simulink model "multi_PMSGs_github"  (R2024a)
settings: Solver=ode1  StartTime=0.0  StopTime=0.5  RelTol=1e-3  EnableMultiTasking=on
libraries: spsCurrentMeasurementLib x3, spsVoltageMeasurementLib x3, spsSeriesRLCBranchLib x2, eeGeneralControl x2, simulink x2, spsdq0toabcLib x2, spsPermanentMagnetSynchronousMachineLib x2, spsUniversalBridgeLib x2, spsGroundLib x1, sps_lib x1
settings Model: Creator=Ruochen Zhao  LastModifiedBy=赵若辰
settings SolverCC: AllowMultiTaskInputOutput=on  PositivePriorityOrder=on  AutoInsertRateTranBlk=on

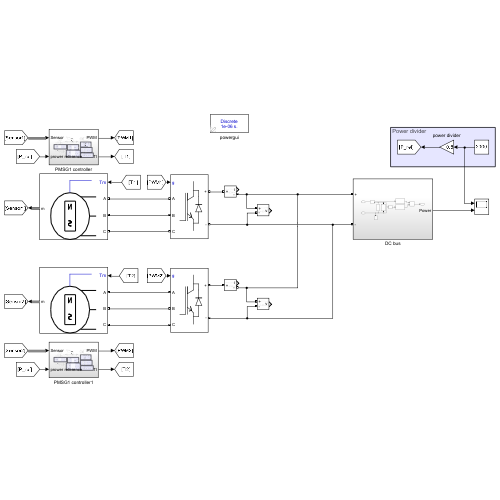
[thumbnail: Simulink's stored preview of the top-level diagram]
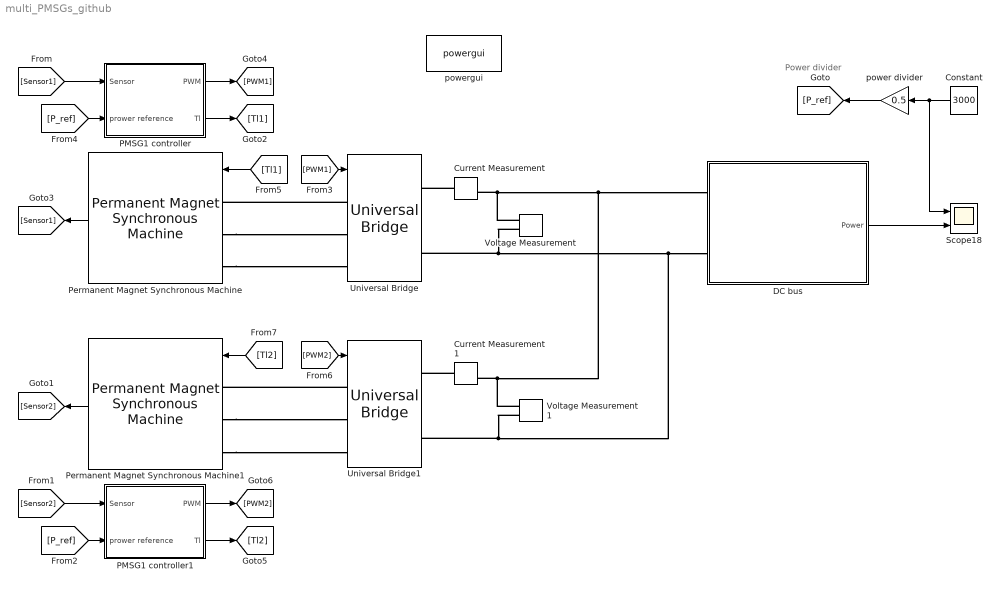
== system multi_PMSGs_github ==
  note: Power divider
  Constant : Constant  Value=3000
  Current Measurement : spsCurrentMeasurementLib/Current Measurement  PhasorSimulation=off  OutputType=Complex  PSBequivalent=0
  Current Measurement1 : spsCurrentMeasurementLib/Current Measurement  PhasorSimulation=off  OutputType=Complex  PSBequivalent=0
  DC bus : Subsystem
  PMSG1 controller : Subsystem
  PMSG1 controller1 : Subsystem
  Permanent Magnet Synchronous Machine : spsPermanentMagnetSynchronousMachineLib/Permanent Magnet Synchronous Machine  NbPhases=3  FluxDistribution=Sinusoidal  RotorType=Salient-pole  MechanicalLoad=Torque Tm  PresetModel=No  ShowDetailedParameters=on  MeasurementBus=off  Resistance=1.3  Inductance=8.5e-3  dqInductances=[0.75e-3,0.75e-3]  La=0.75e-3  MachineConstant=Flux linkage established by magnets (V.s)  Flux=0.4  VoltageCst=145.1039  TorqueCst=1.2  Flat=120  Mechanical="[0.0008 0.00001  2 0 ]"  PolePairs=4  InitialConditions=[0,0, 0,0]  InitialConditions5ph=[0 0 0 0 0 0]  RefAngle=90 degrees behind phase A axis (modified Park)  IterativeDiscreteModel=Trapezoidal non iterative  TsBlock=-1  TsPowergui=0
  Permanent Magnet Synchronous Machine1 : spsPermanentMagnetSynchronousMachineLib/Permanent Magnet Synchronous Machine  NbPhases=3  FluxDistribution=Sinusoidal  RotorType=Salient-pole  MechanicalLoad=Torque Tm  PresetModel=No  ShowDetailedParameters=on  MeasurementBus=off  Resistance=1.3  Inductance=8.5e-3  dqInductances=[0.75e-3,0.75e-3]  La=0.75e-3  MachineConstant=Flux linkage established by magnets (V.s)  Flux=0.4  VoltageCst=145.1039  TorqueCst=1.2  Flat=120  Mechanical="[0.0008 0.00001  2 0 ]"  PolePairs=4  InitialConditions=[0,0, 0,0]  InitialConditions5ph=[0 0 0 0 0 0]  RefAngle=90 degrees behind phase A axis (modified Park)  IterativeDiscreteModel=Trapezoidal non iterative  TsBlock=-1  TsPowergui=0
  Scope18 : Scope  NumInputPorts=2
  Universal Bridge : spsUniversalBridgeLib/Universal Bridge  Arms=3  SnubberResistance=1e5  SnubberCapacitance=inf  Device=IGBT / Diodes  Ron=1e-3  Lon=0  ForwardVoltages="[  0  0  ]"  ForwardVoltage=0  GTOparameters=[ 10e-6 , 20e-6 ]  IGBTparameters=[ 1e-6 , 2e-6 ]  Measurements=None  Measurements_2=None  converterType=Rectifier
  Universal Bridge1 : spsUniversalBridgeLib/Universal Bridge  Arms=3  SnubberResistance=1e5  SnubberCapacitance=inf  Device=IGBT / Diodes  Ron=1e-3  Lon=0  ForwardVoltages="[  0  0  ]"  ForwardVoltage=0  GTOparameters=[ 10e-6 , 20e-6 ]  IGBTparameters=[ 1e-6 , 2e-6 ]  Measurements=None  Measurements_2=None  converterType=Rectifier
  Voltage Measurement : spsVoltageMeasurementLib/Voltage Measurement  PhasorSimulation=off  OutputType=Complex  PSBequivalent=0
  Voltage Measurement1 : spsVoltageMeasurementLib/Voltage Measurement  PhasorSimulation=off  OutputType=Complex  PSBequivalent=0
  power divider : Gain  Gain=0.5
  powergui : sps_lib/powergui  Priority=1  SimulationMode=Discrete  SampleTime=1e-6  frequency=60  Iterations=50  frequencyindice=0  Pbase=100e6  ErrMax=1e-4  UnitsV=kV  UnitsW=MW  buscounter=0  FunctionMessages=off  echomessages=off  EnableUseOfTLC=off  CurrentSourceSwitches=off  DisableSnubberDevices=off  DisableRonSwitches=off  DisableVfSwitches=off  DisplayEquations=off  AutomaticDiscreteSolvers=off  SolverType=Tustin/Backward Euler (TBE)  Interpol=off  ExternalGateDelay=off  methode=off  Ts=100  x0status=blocks  SPID=on  SwTol=0  HookPort=off  NonlinearTolerance=1e-4  nMaxIteration=100  ContinueOnMaxIteration=off  RestoreLinks=warning  ResistiveCurrentMeasurement=off  Frange=[0:2:500]  Ylog=off  Xlog=on  ShowGrid=off  save=off  variable=ZData  structure=0  ZoomFFT=off  StartTime=0.0  cycles=1  DisplayStyle=1  fundamental=60  FreqAxis=off  MaxFrequency=1000  frequencyindicesteady=1  RmsSteady=1  display=off
  wires:
  Permanent Magnet Synchronous Machine/1 -> [Sensor1]
  [Tl1] -> Permanent Magnet Synchronous Machine/1
  [PWM1] -> Universal Bridge/1
  Permanent Magnet Synchronous Machine1/1 -> [Sensor2]
  [PWM2] -> Universal Bridge1/1
  [Sensor1] -> PMSG1 controller/1(Sensor)
  [P_ref] -> PMSG1 controller/2(prower reference)
  Constant/1 -> Scope18/1, power divider/1
  power divider/1 -> [P_ref]
  DC bus/1(Power) -> Scope18/2
  PMSG1 controller/2(Tl) -> [Tl1]
  PMSG1 controller/1(PWM) -> [PWM1]
  PMSG1 controller1/1(PWM) -> [PWM2]
  [P_ref] -> PMSG1 controller1/2(prower reference)
  [Sensor2] -> PMSG1 controller1/1(Sensor)
  PMSG1 controller1/2(Tl) -> [Tl2]
  [Tl2] -> Permanent Magnet Synchronous Machine1/1
  connections:
  Current Measurement1/RConn1 -- DC bus/LConn1 -- Voltage Measurement/LConn1 -- Current Measurement/RConn1 -- Voltage Measurement1/LConn1
  Universal Bridge1/RConn2 -- DC bus/LConn2 -- Voltage Measurement/LConn2 -- Universal Bridge/RConn2 -- Voltage Measurement1/LConn2
  Current Measurement/LConn1 -- Universal Bridge/RConn1
  Permanent Magnet Synchronous Machine/LConn3 -- Universal Bridge/LConn3
  Permanent Magnet Synchronous Machine/LConn2 -- Universal Bridge/LConn2
  Universal Bridge/LConn1 -- Permanent Magnet Synchronous Machine/LConn1
  Current Measurement1/LConn1 -- Universal Bridge1/RConn1
  Permanent Magnet Synchronous Machine1/LConn3 -- Universal Bridge1/LConn3
  Permanent Magnet Synchronous Machine1/LConn2 -- Universal Bridge1/LConn2
  Universal Bridge1/LConn1 -- Permanent Magnet Synchronous Machine1/LConn1

== system multi_PMSGs_github/DC bus ==
  Current Measurement : spsCurrentMeasurementLib/Current Measurement  PhasorSimulation=off  OutputType=Complex  PSBequivalent=0
  Ground : spsGroundLib/Ground  LConnTagsString=a
  Product : Product
  Series RLC Branch : spsSeriesRLCBranchLib/Series RLC Branch  LConnTagsString=__new0  RConnTagsString=__new0  BranchType=R  Resistance=10  Inductance=1e-3  SetiL0=off  InitialCurrent=0  Capacitance=200e-6  Setx0=off  InitialVoltage=0  Measurements=None
  Series RLC Branch1 : spsSeriesRLCBranchLib/Series RLC Branch  LConnTagsString=__new0  RConnTagsString=__new0  BranchType=C  Resistance=50  Inductance=1e-3  SetiL0=off  InitialCurrent=0  Capacitance=200e-6  Setx0=off  InitialVoltage=0  Measurements=None
  Transfer Fcn : TransferFcn  Numerator=[100]  Denominator=[1 100]
  Transfer Fcn1 : TransferFcn  Numerator=[100]  Denominator=[1 100]
  Voltage Measurement : spsVoltageMeasurementLib/Voltage Measurement  PhasorSimulation=off  OutputType=Complex  PSBequivalent=0
  + : PMIOPort  Side=Left
  - : PMIOPort  Port=2  Side=Left
  Power : Outport
  wires:
  Current Measurement/1 -> Transfer Fcn/1
  Transfer Fcn/1 -> Product/1
  Product/1 -> Power/1
  Voltage Measurement/1 -> Transfer Fcn1/1
  Transfer Fcn1/1 -> Product/2
  connections:
  Ground/LConn1 -- -/RConn1 -- Series RLC Branch1/RConn1 -- Voltage Measurement/LConn2 -- Series RLC Branch/RConn1
  Series RLC Branch/LConn1 -- Series RLC Branch1/LConn1 -- Voltage Measurement/LConn1 -- Current Measurement/RConn1
  Current Measurement/LConn1 -- +/RConn1

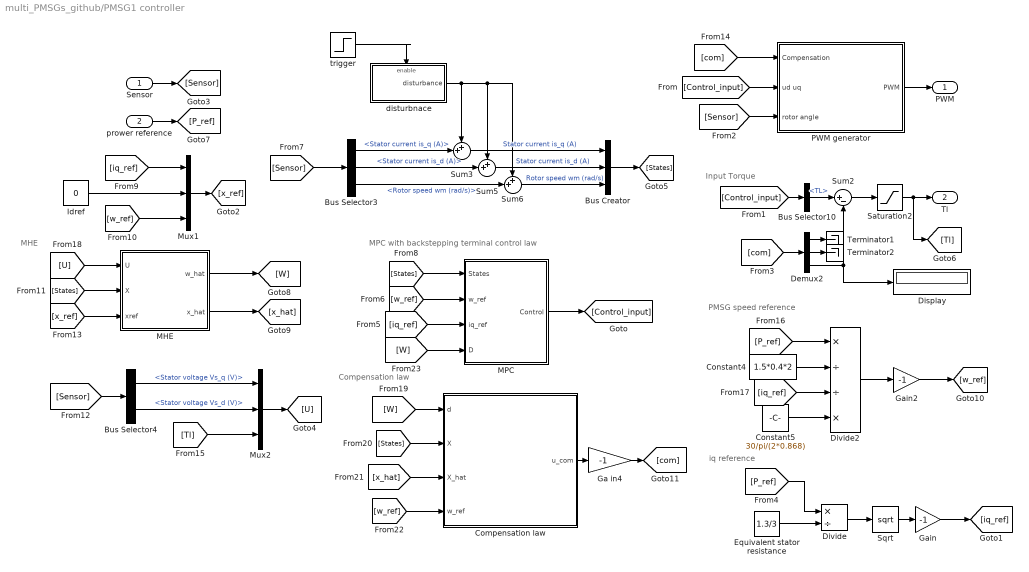
== system multi_PMSGs_github/PMSG1 controller ==
  note: MHE
  note: Compensation law
  note: iq reference
  note: PMSG speed reference
  note: MPC with backstepping terminal control law
  note: Input Torque
  Sensor : Inport
  prower reference : Inport  Port=2
  Bus Creator : BusCreator  Inputs=Stator current is_q (A),Stator current is_d (A),Rotor speed wm (rad/s)
  Bus Selector10 : BusSelector  OutputSignals=TL
  Bus Selector3 : BusSelector  OutputSignals=Stator current is_q (A),Stator current is_d (A),Rotor speed wm (rad/s)
  Bus Selector4 : BusSelector  OutputSignals=Stator voltage Vs_q (V),Stator voltage Vs_d (V)
  Compensation law : Subsystem  mask{K1=10000*10, K2=10000*6, K3=0}
      mask DialogControl ParameterGroupVar Prompt: 参数
  Constant4 : Constant  Value=1.5*0.4*2
  Constant5 : Constant  Value=30/pi/(2*0.868)
  Demux2 : Demux  Outputs=3
  Display : Display
  Divide : Product  Inputs=*/
  Divide2 : Product  Inputs=*//*
  Equivalent stator resistance : Constant  Value=1.3/3
  Ga in4 : Gain  Gain=-1
  Gain : Gain  Gain=-1
  Gain2 : Gain  Gain=-1
  Idref : Constant  Value=0
  MHE : Subsystem
  MPC : Subsystem  mask{q1=100, q2=100, q3=100, r1=0.01, r2=0.001, r3=0.001, N=10, K1=1e5*0.1, K2=1e5*0.1, K3=1e5*0.1, fc=100, Ts=1e-5}
      mask DialogControl DescGroupVar Prompt: MPC controller
      mask DialogControl ParameterGroupVar Prompt: Output Weight
      mask DialogControl Container3 Prompt: Input Weight
      mask DialogControl Container4 Prompt: Prediction Horizon
      mask DialogControl Container5 Prompt: Backstepping
      mask DialogControl Container6 Prompt: Filter
      mask DialogControl Container7 Prompt: Simple Time
  Mux1 : Mux  Inputs=3
  Mux2 : Mux  Inputs=3
  PWM generator : Subsystem
  Saturation2 : Saturate  UpperLimit=300  LowerLimit=-300
  Sqrt : Sqrt
  Sum2 : Sum  Inputs=|+-
  Sum3 : Sum  Inputs=++|
  Sum5 : Sum  Inputs=++|
  Sum6 : Sum  Inputs=++|
  Terminator1 : Terminator
  Terminator2 : Terminator
  disturbnace : Subsystem  mask{w1=50, A1=5, w2=100, A2=2, w3=150, A3=1}
      mask prompts: w1 "Frequency 1"; A1 "Amplitude 1"; w2 "Frequency 2"; A2 "Amplitude 2"; w3 "Frequency 3"; A3 "Amplitude 3"
      mask DialogControl ParameterGroupVar Prompt: 参数
  trigger : Step  Time=0.2  SampleTime=0
  PWM : Outport
  Tl : Outport  Port=2
  wires:
  Sensor/1 -> [Sensor]
  MPC/1(Control) -> [Control_input]
  [Control_input] -> Bus Selector10/1
  Bus Selector10/1 -> Sum2/1  "<TL>"
  Sum2/1 -> Saturation2/1
  [com] -> Demux2/1
  Demux2/3 -> Sum2/2, Display/1
  Demux2/1 -> Terminator1/1
  Demux2/2 -> Terminator2/1
  prower reference/1 -> [P_ref]
  Divide/1 -> Sqrt/1
  Equivalent stator resistance/1 -> Divide/2
  Sqrt/1 -> Gain/1
  [P_ref] -> Divide/1
  Gain/1 -> [iq_ref]
  [iq_ref] -> MPC/3(iq_ref)
  Bus Selector3/3 -> Sum6/2  "<Rotor speed wm (rad/s)>"
  Sum5/1 -> Bus Creator/2  "Stator current is_d (A)"
  Sum3/1 -> Bus Creator/1  "Stator current is_q (A)"
  Sum6/1 -> Bus Creator/3  "Rotor speed wm (rad/s)"
  Bus Selector3/1 -> Sum3/2  "<Stator current is_q (A)>"
  [Sensor] -> Bus Selector3/1
  Bus Selector3/2 -> Sum5/2  "<Stator current is_d (A)>"
  Bus Creator/1 -> [States]
  [com] -> PWM generator/1(Compensation)
  [Control_input] -> PWM generator/2(ud uq)
  [Sensor] -> PWM generator/3(rotor angle)
  PWM generator/1(PWM) -> PWM/1
  [iq_ref] -> Divide2/3
  Constant5/1 -> Divide2/4
  Gain2/1 -> [w_ref]
  Divide2/1 -> Gain2/1
  [P_ref] -> Divide2/1
  Constant4/1 -> Divide2/2
  [w_ref] -> MPC/2(w_ref)
  [States] -> MPC/1(States)
  disturbnace/1(disturbance) -> Sum6/1, Sum5/1, Sum3/1
  trigger/1 -> disturbnace/Enable
  [iq_ref] -> Mux1/1
  Idref/1 -> Mux1/2
  [w_ref] -> Mux1/3
  Mux1/1 -> [x_ref]
  [Tl] -> Mux2/3
  [Sensor] -> Bus Selector4/1
  Bus Selector4/2 -> Mux2/2  "<Stator voltage Vs_d (V)>"
  Mux2/1 -> [U]
  Bus Selector4/1 -> Mux2/1  "<Stator voltage Vs_q (V)>"
  [U] -> MHE/1("U ")
  [States] -> MHE/2(X)
  [x_ref] -> MHE/3(xref)
  MHE/1(w_hat) -> [W]
  [W] -> Compensation law/1(d)
  [States] -> Compensation law/2(X)
  MHE/2(x_hat) -> [x_hat]
  [x_hat] -> Compensation law/3(X_hat)
  [w_ref] -> Compensation law/4(w_ref)
  Ga in4/1 -> [com]
  Compensation law/1(u_com) -> Ga in4/1
  [W] -> MPC/4(D)
  Saturation2/1 -> [Tl], Tl/1

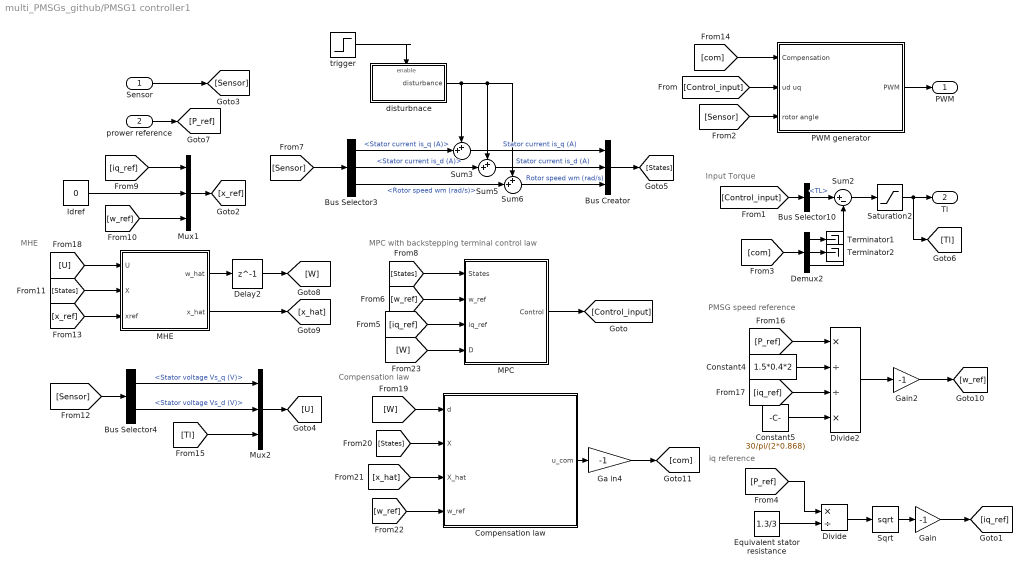
== system multi_PMSGs_github/PMSG1 controller1 ==
  note: MHE
  note: Compensation law
  note: iq reference
  note: PMSG speed reference
  note: MPC with backstepping terminal control law
  note: Input Torque
  Sensor : Inport
  prower reference : Inport  Port=2
  Bus Creator : BusCreator  Inputs=Stator current is_q (A),Stator current is_d (A),Rotor speed wm (rad/s)
  Bus Selector10 : BusSelector  OutputSignals=TL
  Bus Selector3 : BusSelector  OutputSignals=Stator current is_q (A),Stator current is_d (A),Rotor speed wm (rad/s)
  Bus Selector4 : BusSelector  OutputSignals=Stator voltage Vs_q (V),Stator voltage Vs_d (V)
  Compensation law : Subsystem  mask{K1=10000*10, K2=10000*6, K3=0}
      mask DialogControl ParameterGroupVar Prompt: 参数
  Constant4 : Constant  Value=1.5*0.4*2
  Constant5 : Constant  Value=30/pi/(2*0.868)
  Delay2 : Delay  DelayLength=1  InitialCondition=[0 0 0]
  Demux2 : Demux  Outputs=3
  Divide : Product  Inputs=*/
  Divide2 : Product  Inputs=*//*
  Equivalent stator resistance : Constant  Value=1.3/3
  Ga in4 : Gain  Gain=-1
  Gain : Gain  Gain=-1
  Gain2 : Gain  Gain=-1
  Idref : Constant  Value=0
  MHE : Subsystem
  MPC : Subsystem  mask{q1=100, q2=100, q3=100, r1=0.01, r2=0.001, r3=0.001, N=10, K1=1e5*0.1, K2=1e5*0.1, K3=1e5*0.1, fc=100, Ts=1e-5}
      mask DialogControl DescGroupVar Prompt: MPC controller
      mask DialogControl ParameterGroupVar Prompt: Output Weight
      mask DialogControl Container3 Prompt: Input Weight
      mask DialogControl Container4 Prompt: Prediction Horizon
      mask DialogControl Container5 Prompt: Backstepping
      mask DialogControl Container6 Prompt: Filter
      mask DialogControl Container7 Prompt: Simple Time
  Mux1 : Mux  Inputs=3
  Mux2 : Mux  Inputs=3
  PWM generator : Subsystem
  Saturation2 : Saturate  UpperLimit=300  LowerLimit=-300
  Sqrt : Sqrt
  Sum2 : Sum  Inputs=|+-
  Sum3 : Sum  Inputs=++|
  Sum5 : Sum  Inputs=++|
  Sum6 : Sum  Inputs=++|
  Terminator1 : Terminator
  Terminator2 : Terminator
  disturbnace : Subsystem  mask{w1=50, A1=5, w2=100, A2=2, w3=150, A3=1}
      mask prompts: w1 "Frequency 1"; A1 "Amplitude 1"; w2 "Frequency 2"; A2 "Amplitude 2"; w3 "Frequency 3"; A3 "Amplitude 3"
      mask DialogControl ParameterGroupVar Prompt: 参数
  trigger : Step  Time=0.2  After=0  SampleTime=0
  PWM : Outport
  Tl : Outport  Port=2
  wires:
  Sensor/1 -> [Sensor]
  MPC/1(Control) -> [Control_input]
  [Control_input] -> Bus Selector10/1
  Bus Selector10/1 -> Sum2/1  "<TL>"
  Sum2/1 -> Saturation2/1
  [com] -> Demux2/1
  Demux2/3 -> Sum2/2
  Demux2/1 -> Terminator1/1
  Demux2/2 -> Terminator2/1
  prower reference/1 -> [P_ref]
  Divide/1 -> Sqrt/1
  Equivalent stator resistance/1 -> Divide/2
  Sqrt/1 -> Gain/1
  [P_ref] -> Divide/1
  Gain/1 -> [iq_ref]
  [iq_ref] -> MPC/3(iq_ref)
  Bus Selector3/3 -> Sum6/2  "<Rotor speed wm (rad/s)>"
  Sum5/1 -> Bus Creator/2  "Stator current is_d (A)"
  Sum3/1 -> Bus Creator/1  "Stator current is_q (A)"
  Sum6/1 -> Bus Creator/3  "Rotor speed wm (rad/s)"
  Bus Selector3/1 -> Sum3/2  "<Stator current is_q (A)>"
  [Sensor] -> Bus Selector3/1
  Bus Selector3/2 -> Sum5/2  "<Stator current is_d (A)>"
  Bus Creator/1 -> [States]
  [com] -> PWM generator/1(Compensation)
  [Control_input] -> PWM generator/2(ud uq)
  [Sensor] -> PWM generator/3(rotor angle)
  PWM generator/1(PWM) -> PWM/1
  [iq_ref] -> Divide2/3
  Constant5/1 -> Divide2/4
  Gain2/1 -> [w_ref]
  Divide2/1 -> Gain2/1
  [P_ref] -> Divide2/1
  Constant4/1 -> Divide2/2
  [w_ref] -> MPC/2(w_ref)
  [States] -> MPC/1(States)
  disturbnace/1(disturbance) -> Sum6/1, Sum5/1, Sum3/1
  trigger/1 -> disturbnace/Enable
  [iq_ref] -> Mux1/1
  Idref/1 -> Mux1/2
  [w_ref] -> Mux1/3
  Mux1/1 -> [x_ref]
  [Tl] -> Mux2/3
  [Sensor] -> Bus Selector4/1
  Bus Selector4/2 -> Mux2/2  "<Stator voltage Vs_d (V)>"
  Mux2/1 -> [U]
  Bus Selector4/1 -> Mux2/1  "<Stator voltage Vs_q (V)>"
  [U] -> MHE/1("U ")
  [States] -> MHE/2(X)
  [x_ref] -> MHE/3(xref)
  MHE/1(w_hat) -> Delay2/1
  Delay2/1 -> [W]
  [W] -> Compensation law/1(d)
  [States] -> Compensation law/2(X)
  MHE/2(x_hat) -> [x_hat]
  [x_hat] -> Compensation law/3(X_hat)
  [w_ref] -> Compensation law/4(w_ref)
  Ga in4/1 -> [com]
  Compensation law/1(u_com) -> Ga in4/1
  [W] -> MPC/4(D)
  Saturation2/1 -> [Tl], Tl/1

== system multi_PMSGs_github/PMSG1 controller/Compensation law ==
  d : Inport
  X : Inport  Port=2
  X_hat : Inport  Port=3
  w_ref : Inport  Port=4
  Constant : Constant  Value=K1
  Constant1 : Constant  Value=K2
  Constant2 : Constant  Value=K3
  MATLAB Function : MATLAB Function  TreatAsAtomicUnit=on
  u_com : Outport
  wires:
  Constant2/1 -> MATLAB Function/4(K3)
  Constant/1 -> MATLAB Function/2(K1)
  Constant1/1 -> MATLAB Function/3(K2)
  MATLAB Function/1(u_com) -> u_com/1
  d/1 -> MATLAB Function/1(w)
  X/1 -> MATLAB Function/5(X)
  X_hat/1 -> MATLAB Function/6(X_hat)
  w_ref/1 -> MATLAB Function/7(w_ref)

== system multi_PMSGs_github/PMSG1 controller/MHE ==
  "U " : Inport
  X : Inport  Port=2
  xref : Inport  Port=3
  Delay1 : Delay  DelayLength=1  InitialCondition=[0 0 0].'
  Delay2 : Delay  DelayLength=1  InitialCondition=[0 0 0]
  MATLAB Function1 : MATLAB Function  TreatAsAtomicUnit=on
  MHE1 : Subsystem
  w_hat : Outport
  x_hat : Outport  Port=2
  wires:
  X/1 -> MHE1/2(X)
  MHE1/1(y) -> Delay2/1
  xref/1 -> MHE1/3(xref)
  "U "/1 -> MATLAB Function1/2(u), MHE1/1("U ")
  MATLAB Function1/1(xk_dot) -> Delay1/1
  Delay1/1 -> x_hat/1, MATLAB Function1/1(xk), MHE1/4(xk)
  Delay2/1 -> w_hat/1

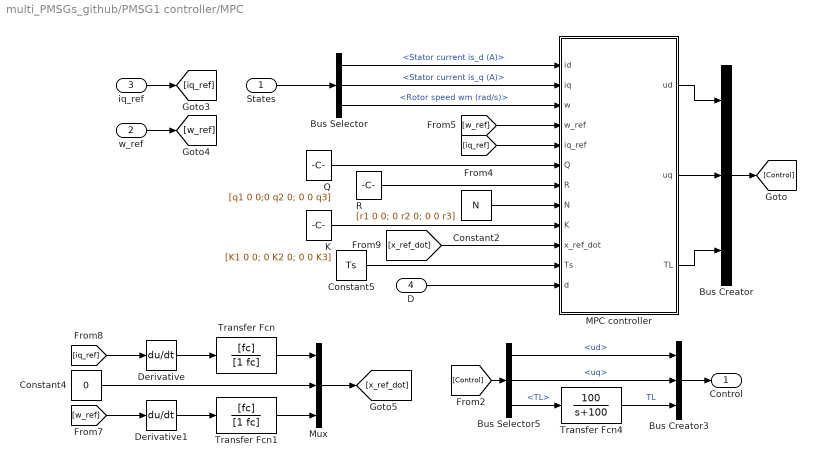
== system multi_PMSGs_github/PMSG1 controller/MPC ==
  States : Inport
  w_ref : Inport  Port=2
  iq_ref : Inport  Port=3
  D : Inport  Port=4
  Bus Creator : BusCreator  Inputs=3
  Bus Creator3 : BusCreator  Inputs=3
  Bus Selector : BusSelector  OutputSignals=Stator current is_d (A),Stator current is_q (A),Rotor speed wm (rad/s)
  Bus Selector5 : BusSelector  OutputSignals=ud,uq,TL
  Constant2 : Constant  Value=N
  Constant4 : Constant  Value=0
  Constant5 : Constant  Value=Ts
  Derivative : Derivative
  Derivative1 : Derivative
  K : Constant  Value=[K1 0 0; 0 K2 0; 0 0 K3]
  "MPC controller " : MATLAB Function  TreatAsAtomicUnit=on
  Mux : Mux  Inputs=3
  Q : Constant  Value=[q1 0 0;0 q2 0; 0 0 q3]
  R : Constant  Value=[r1 0 0; 0 r2 0; 0 0 r3]
  Transfer Fcn : TransferFcn  Numerator=[fc]  Denominator=[1 fc]
  Transfer Fcn1 : TransferFcn  Numerator=[fc]  Denominator=[1 fc]
  Transfer Fcn4 : TransferFcn  Numerator=[100]  Denominator=[1 100]
  Control : Outport
  wires:
  Bus Selector/3 -> "MPC controller "/3(w)  "<Rotor speed wm (rad/s)>"
  Bus Selector/1 -> "MPC controller "/1(id)  "<Stator current is_d (A)>"
  Bus Selector/2 -> "MPC controller "/2(iq)  "<Stator current is_q (A)>"
  "MPC controller "/2(uq) -> Bus Creator/2
  "MPC controller "/1(ud) -> Bus Creator/1
  "MPC controller "/3(TL) -> Bus Creator/3
  Bus Creator/1 -> [Control]
  States/1 -> Bus Selector/1
  [Control] -> Bus Selector5/1
  Bus Selector5/1 -> Bus Creator3/1  "<ud>"
  Bus Selector5/3 -> Transfer Fcn4/1  "<TL>"
  Bus Selector5/2 -> Bus Creator3/2  "<uq>"
  Transfer Fcn4/1 -> Bus Creator3/3  "TL"
  Bus Creator3/1 -> Control/1
  Q/1 -> "MPC controller "/6(Q)
  R/1 -> "MPC controller "/7(R)
  Constant2/1 -> "MPC controller "/8(N)
  K/1 -> "MPC controller "/9(K)
  iq_ref/1 -> [iq_ref]
  w_ref/1 -> [w_ref]
  [iq_ref] -> "MPC controller "/5(iq_ref)
  [w_ref] -> "MPC controller "/4(w_ref)
  Constant4/1 -> Mux/2
  [iq_ref] -> Derivative/1
  Derivative/1 -> Transfer Fcn/1
  [w_ref] -> Derivative1/1
  Derivative1/1 -> Transfer Fcn1/1
  Transfer Fcn/1 -> Mux/1
  Transfer Fcn1/1 -> Mux/3
  Mux/1 -> [x_ref_dot]
  [x_ref_dot] -> "MPC controller "/10(x_ref_dot)
  Constant5/1 -> "MPC controller "/11(Ts)
  D/1 -> "MPC controller "/12(d)

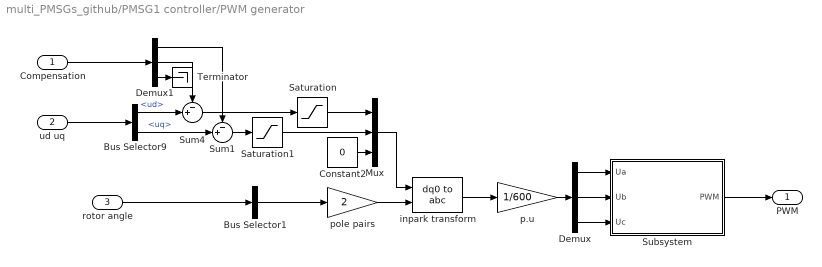
== system multi_PMSGs_github/PMSG1 controller/PWM generator ==
  Compensation : Inport
  ud uq : Inport  Port=2
  rotor angle : Inport  Port=3
  Bus Selector1 : BusSelector  OutputSignals=Rotor angle thetam (rad)  OutputAsBus=on
  Bus Selector9 : BusSelector  OutputSignals=ud,uq
  Constant2 : Constant  Value=0
  Demux : Demux  Outputs=3
  Demux1 : Demux  Outputs=3
  Mux : Mux  Inputs=3
  Saturation : Saturate  UpperLimit=600  LowerLimit=-600
  Saturation1 : Saturate  UpperLimit=600  LowerLimit=-600
  Subsystem : Subsystem
  Sum1 : Sum  Inputs=-+|
  Sum4 : Sum  Inputs=-+|
  Terminator : Terminator
  inpark transform : spsdq0toabcLib/dq0 to abc  Alignment=Aligned with phase A axis
  p.u : Gain  Gain=1/600
  pole pairs : Gain  Gain=2
  PWM : Outport
  wires:
  Mux/1 -> inpark transform/1
  p.u/1 -> Demux/1
  Bus Selector1/1 -> pole pairs/1
  Constant2/1 -> Mux/3
  Demux1/1 -> Sum1/1
  Sum4/1 -> Saturation/1
  Bus Selector9/1 -> Sum4/2  "<ud>"
  pole pairs/1 -> inpark transform/2
  Demux/2 -> Subsystem/2(Ub)
  rotor angle/1 -> Bus Selector1/1
  Demux/3 -> Subsystem/3(Uc)
  Demux/1 -> Subsystem/1(Ua)
  inpark transform/1 -> p.u/1
  Sum1/1 -> Saturation1/1
  Demux1/3 -> Terminator/1
  Bus Selector9/2 -> Sum1/2  "<uq>"
  Demux1/2 -> Sum4/1
  Subsystem/1(PWM) -> PWM/1
  ud uq/1 -> Bus Selector9/1
  Compensation/1 -> Demux1/1
  Saturation/1 -> Mux/1
  Saturation1/1 -> Mux/2

== system multi_PMSGs_github/PMSG1 controller/disturbnace ==
  Enable : EnablePort
  Sine Wave : Sin  Amplitude=A1  Frequency=w1*2*pi  SampleTime=0
  Sine Wave1 : Sin  Amplitude=A2  Frequency=w2*2*pi  SampleTime=0
  Sine Wave2 : Sin  Amplitude=A3  Frequency=w3*2*pi  SampleTime=0
  Sum : Sum  Inputs=+++
  disturbance : Outport
  wires:
  Sine Wave1/1 -> Sum/2
  Sine Wave/1 -> Sum/1
  Sine Wave2/1 -> Sum/3
  Sum/1 -> disturbance/1

== system multi_PMSGs_github/PMSG1 controller1/Compensation law ==
  d : Inport
  X : Inport  Port=2
  X_hat : Inport  Port=3
  w_ref : Inport  Port=4
  Constant : Constant  Value=K1
  Constant1 : Constant  Value=K2
  Constant2 : Constant  Value=K3
  MATLAB Function : MATLAB Function  TreatAsAtomicUnit=on
  u_com : Outport
  wires:
  Constant2/1 -> MATLAB Function/4(K3)
  Constant/1 -> MATLAB Function/2(K1)
  Constant1/1 -> MATLAB Function/3(K2)
  MATLAB Function/1(u_com) -> u_com/1
  d/1 -> MATLAB Function/1(w)
  X/1 -> MATLAB Function/5(X)
  X_hat/1 -> MATLAB Function/6(X_hat)
  w_ref/1 -> MATLAB Function/7(w_ref)

== system multi_PMSGs_github/PMSG1 controller1/MHE ==
  "U " : Inport
  X : Inport  Port=2
  xref : Inport  Port=3
  Delay1 : Delay  DelayLength=1  InitialCondition=[0 0 0].'
  MATLAB Function1 : MATLAB Function  TreatAsAtomicUnit=on
  MHE1 : Subsystem
  w_hat : Outport
  x_hat : Outport  Port=2
  wires:
  X/1 -> MHE1/2(X)
  MHE1/1(y) -> w_hat/1
  xref/1 -> MHE1/3(xref)
  "U "/1 -> MATLAB Function1/2(u), MHE1/1("U ")
  MATLAB Function1/1(xk_dot) -> Delay1/1
  Delay1/1 -> x_hat/1, MATLAB Function1/1(xk), MHE1/4(xk)

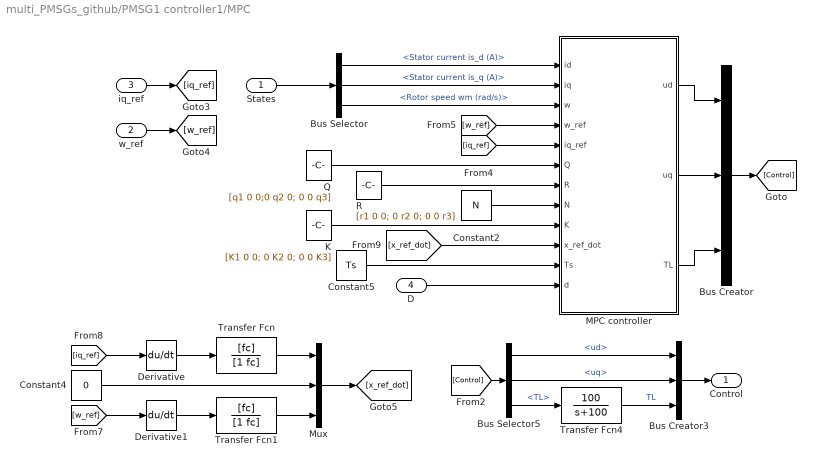
== system multi_PMSGs_github/PMSG1 controller1/MPC ==
  States : Inport
  w_ref : Inport  Port=2
  iq_ref : Inport  Port=3
  D : Inport  Port=4
  Bus Creator : BusCreator  Inputs=3
  Bus Creator3 : BusCreator  Inputs=3
  Bus Selector : BusSelector  OutputSignals=Stator current is_d (A),Stator current is_q (A),Rotor speed wm (rad/s)
  Bus Selector5 : BusSelector  OutputSignals=ud,uq,TL
  Constant2 : Constant  Value=N
  Constant4 : Constant  Value=0
  Constant5 : Constant  Value=Ts
  Derivative : Derivative
  Derivative1 : Derivative
  K : Constant  Value=[K1 0 0; 0 K2 0; 0 0 K3]
  "MPC controller " : MATLAB Function  TreatAsAtomicUnit=on
  Mux : Mux  Inputs=3
  Q : Constant  Value=[q1 0 0;0 q2 0; 0 0 q3]
  R : Constant  Value=[r1 0 0; 0 r2 0; 0 0 r3]
  Transfer Fcn : TransferFcn  Numerator=[fc]  Denominator=[1 fc]
  Transfer Fcn1 : TransferFcn  Numerator=[fc]  Denominator=[1 fc]
  Transfer Fcn4 : TransferFcn  Numerator=[100]  Denominator=[1 100]
  Control : Outport
  wires:
  Bus Selector/3 -> "MPC controller "/3(w)  "<Rotor speed wm (rad/s)>"
  Bus Selector/1 -> "MPC controller "/1(id)  "<Stator current is_d (A)>"
  Bus Selector/2 -> "MPC controller "/2(iq)  "<Stator current is_q (A)>"
  "MPC controller "/2(uq) -> Bus Creator/2
  "MPC controller "/1(ud) -> Bus Creator/1
  "MPC controller "/3(TL) -> Bus Creator/3
  Bus Creator/1 -> [Control]
  States/1 -> Bus Selector/1
  [Control] -> Bus Selector5/1
  Bus Selector5/1 -> Bus Creator3/1  "<ud>"
  Bus Selector5/3 -> Transfer Fcn4/1  "<TL>"
  Bus Selector5/2 -> Bus Creator3/2  "<uq>"
  Transfer Fcn4/1 -> Bus Creator3/3  "TL"
  Bus Creator3/1 -> Control/1
  Q/1 -> "MPC controller "/6(Q)
  R/1 -> "MPC controller "/7(R)
  Constant2/1 -> "MPC controller "/8(N)
  K/1 -> "MPC controller "/9(K)
  iq_ref/1 -> [iq_ref]
  w_ref/1 -> [w_ref]
  [iq_ref] -> "MPC controller "/5(iq_ref)
  [w_ref] -> "MPC controller "/4(w_ref)
  Constant4/1 -> Mux/2
  [iq_ref] -> Derivative/1
  Derivative/1 -> Transfer Fcn/1
  [w_ref] -> Derivative1/1
  Derivative1/1 -> Transfer Fcn1/1
  Transfer Fcn/1 -> Mux/1
  Transfer Fcn1/1 -> Mux/3
  Mux/1 -> [x_ref_dot]
  [x_ref_dot] -> "MPC controller "/10(x_ref_dot)
  Constant5/1 -> "MPC controller "/11(Ts)
  D/1 -> "MPC controller "/12(d)

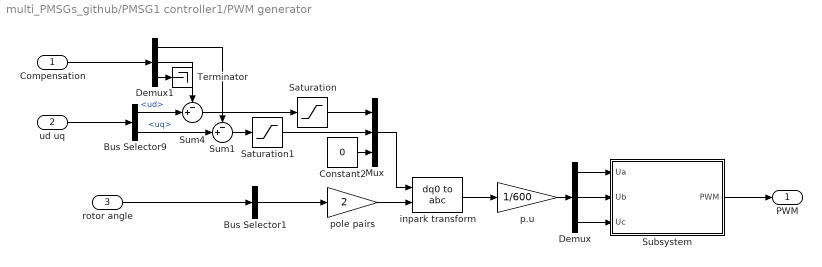
== system multi_PMSGs_github/PMSG1 controller1/PWM generator ==
  Compensation : Inport
  ud uq : Inport  Port=2
  rotor angle : Inport  Port=3
  Bus Selector1 : BusSelector  OutputSignals=Rotor angle thetam (rad)  OutputAsBus=on
  Bus Selector9 : BusSelector  OutputSignals=ud,uq
  Constant2 : Constant  Value=0
  Demux : Demux  Outputs=3
  Demux1 : Demux  Outputs=3
  Mux : Mux  Inputs=3
  Saturation : Saturate  UpperLimit=600  LowerLimit=-600
  Saturation1 : Saturate  UpperLimit=600  LowerLimit=-600
  Subsystem : Subsystem
  Sum1 : Sum  Inputs=-+|
  Sum4 : Sum  Inputs=-+|
  Terminator : Terminator
  inpark transform : spsdq0toabcLib/dq0 to abc  Alignment=Aligned with phase A axis
  p.u : Gain  Gain=1/600
  pole pairs : Gain  Gain=2
  PWM : Outport
  wires:
  Mux/1 -> inpark transform/1
  p.u/1 -> Demux/1
  Bus Selector1/1 -> pole pairs/1
  Constant2/1 -> Mux/3
  Demux1/1 -> Sum1/1
  Sum4/1 -> Saturation/1
  Bus Selector9/1 -> Sum4/2  "<ud>"
  pole pairs/1 -> inpark transform/2
  Demux/2 -> Subsystem/2(Ub)
  rotor angle/1 -> Bus Selector1/1
  Demux/3 -> Subsystem/3(Uc)
  Demux/1 -> Subsystem/1(Ua)
  inpark transform/1 -> p.u/1
  Sum1/1 -> Saturation1/1
  Demux1/3 -> Terminator/1
  Bus Selector9/2 -> Sum1/2  "<uq>"
  Demux1/2 -> Sum4/1
  Subsystem/1(PWM) -> PWM/1
  ud uq/1 -> Bus Selector9/1
  Compensation/1 -> Demux1/1
  Saturation/1 -> Mux/1
  Saturation1/1 -> Mux/2

== system multi_PMSGs_github/PMSG1 controller1/disturbnace ==
  Enable : EnablePort
  Sine Wave : Sin  Amplitude=A1  Frequency=w1*2*pi  SampleTime=0
  Sine Wave1 : Sin  Amplitude=A2  Frequency=w2*2*pi  SampleTime=0
  Sine Wave2 : Sin  Amplitude=A3  Frequency=w3*2*pi  SampleTime=0
  Sum : Sum  Inputs=+++
  disturbance : Outport
  wires:
  Sine Wave1/1 -> Sum/2
  Sine Wave/1 -> Sum/1
  Sine Wave2/1 -> Sum/3
  Sum/1 -> disturbance/1

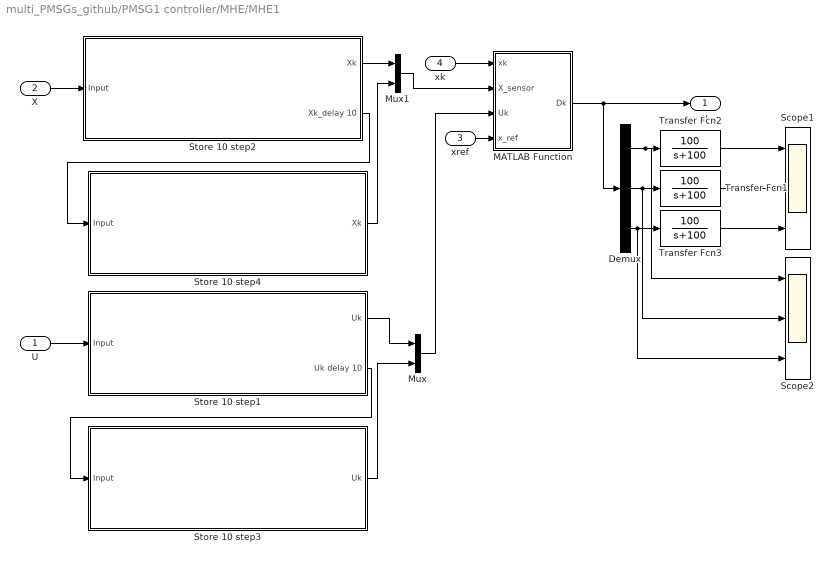
== system multi_PMSGs_github/PMSG1 controller/MHE/MHE1 ==
  "U " : Inport
  X : Inport  Port=2
  xref : Inport  Port=3
  xk : Inport  Port=4
  Demux : Demux  Outputs=3
  MATLAB Function : MATLAB Function  TreatAsAtomicUnit=on
  Mux : Mux  Inputs=2
  Mux1 : Mux  Inputs=2
  Scope1 : Scope  NumInputPorts=3
  Scope2 : Scope  NumInputPorts=3
  Store 10 step1 : Subsystem
  Store 10 step2 : Subsystem
  Store 10 step3 : Subsystem
  Store 10 step4 : Subsystem
  Transfer Fcn1 : TransferFcn  Numerator=[100]  Denominator=[1 100]
  Transfer Fcn2 : TransferFcn  Numerator=[100]  Denominator=[1 100]
  Transfer Fcn3 : TransferFcn  Numerator=[100]  Denominator=[1 100]
  y : Outport
  wires:
  X/1 -> Store 10 step2/1("Input ")
  xref/1 -> MATLAB Function/4(x_ref)
  Demux/2 -> Scope2/2, Transfer Fcn1/1
  Demux/1 -> Scope2/1, Transfer Fcn2/1
  Demux/3 -> Scope2/3, Transfer Fcn3/1
  MATLAB Function/1(Dk) -> Demux/1, y/1
  Transfer Fcn2/1 -> Scope1/1
  Transfer Fcn1/1 -> Scope1/2
  Transfer Fcn3/1 -> Scope1/3
  "U "/1 -> Store 10 step1/1("Input ")
  xk/1 -> MATLAB Function/1(xk)
  Store 10 step1/1(Uk) -> Mux/1
  Store 10 step3/1(Uk) -> Mux/2
  Mux/1 -> MATLAB Function/3(Uk)
  Store 10 step2/2(Xk_delay 10) -> Store 10 step4/1("Input ")
  Store 10 step4/1(Xk) -> Mux1/2
  Store 10 step2/1(Xk) -> Mux1/1
  Mux1/1 -> MATLAB Function/2(X_sensor)
  Store 10 step1/2(Uk delay 10) -> Store 10 step3/1("Input ")

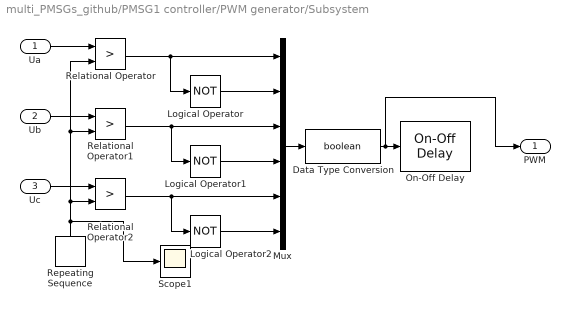
== system multi_PMSGs_github/PMSG1 controller/PWM generator/Subsystem ==
  Ua : Inport
  Ub : Inport  Port=2
  Uc : Inport  Port=3
  Data Type Conversion : DataTypeConversion  OutDataTypeStr=boolean  SaturateOnIntegerOverflow=off  RndMeth=Floor
  Logical Operator : Logic  Operator=NOT  AllPortsSameDT=off  OutDataTypeStr=boolean
  Logical Operator1 : Logic  Operator=NOT  AllPortsSameDT=off  OutDataTypeStr=boolean
  Logical Operator2 : Logic  Operator=NOT  AllPortsSameDT=off  OutDataTypeStr=boolean
  Mux : Mux  Inputs=6
  On-Off Delay : eeGeneralControl/On-Off Delay  LabelModeActiveChoice=Discrete  Td_on=2e-6  Td_off=0  IC=0  Ts=2e-6
      settings: LibrarySourceBlock=ee_sl_lib/General Control/On-Off Delay
  Relational Operator : RelationalOperator  Operator=>  OutDataTypeStr=boolean  RndMeth=Simplest  InputSameDT=off
  Relational Operator1 : RelationalOperator  Operator=>  OutDataTypeStr=boolean  RndMeth=Simplest  InputSameDT=off
  Relational Operator2 : RelationalOperator  Operator=>  OutDataTypeStr=boolean  RndMeth=Simplest  InputSameDT=off
  Repeating Sequence : simulink/Sources/Repeating Sequence  rep_seq_t="[0  (1e-4)/2 1e-4]"  rep_seq_y=[-1 1 -1]
  Scope1 : Scope
  PWM : Outport
  wires:
  Ua/1 -> Relational Operator/1
  Ub/1 -> Relational Operator1/1
  Uc/1 -> Relational Operator2/1
  Repeating Sequence/1 -> Scope1/1, Relational Operator/2, Relational Operator1/2, Relational Operator2/2
  Logical Operator/1 -> Mux/2
  Relational Operator/1 -> Logical Operator/1, Mux/1
  Relational Operator1/1 -> Logical Operator1/1, Mux/3
  Logical Operator1/1 -> Mux/4
  Relational Operator2/1 -> Logical Operator2/1, Mux/5
  Logical Operator2/1 -> Mux/6
  Mux/1 -> Data Type Conversion/1
  Data Type Conversion/1 -> PWM/1, On-Off Delay/1

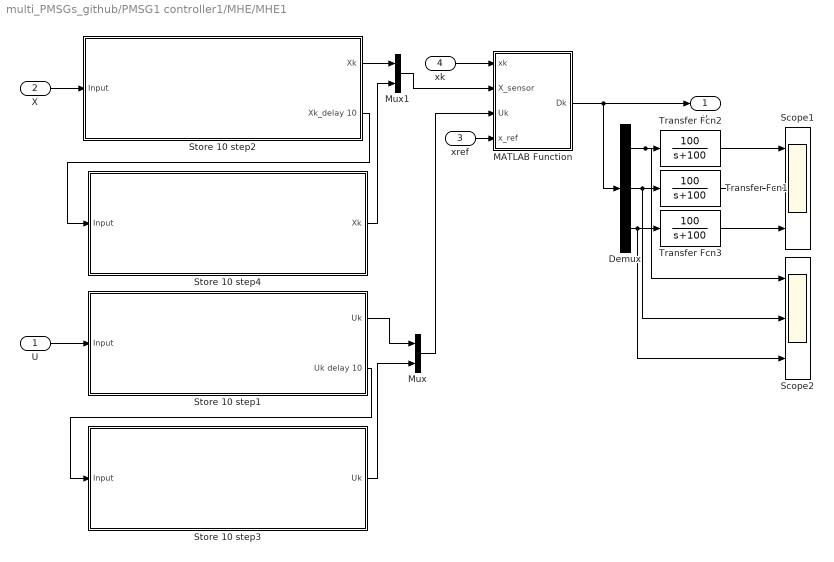
== system multi_PMSGs_github/PMSG1 controller1/MHE/MHE1 ==
  "U " : Inport
  X : Inport  Port=2
  xref : Inport  Port=3
  xk : Inport  Port=4
  Demux : Demux  Outputs=3
  MATLAB Function : MATLAB Function  TreatAsAtomicUnit=on
  Mux : Mux  Inputs=2
  Mux1 : Mux  Inputs=2
  Scope1 : Scope  NumInputPorts=3
  Scope2 : Scope  NumInputPorts=3
  Store 10 step1 : Subsystem
  Store 10 step2 : Subsystem
  Store 10 step3 : Subsystem
  Store 10 step4 : Subsystem
  Transfer Fcn1 : TransferFcn  Numerator=[100]  Denominator=[1 100]
  Transfer Fcn2 : TransferFcn  Numerator=[100]  Denominator=[1 100]
  Transfer Fcn3 : TransferFcn  Numerator=[100]  Denominator=[1 100]
  y : Outport
  wires:
  X/1 -> Store 10 step2/1("Input ")
  xref/1 -> MATLAB Function/4(x_ref)
  Demux/2 -> Scope2/2, Transfer Fcn1/1
  Demux/1 -> Scope2/1, Transfer Fcn2/1
  Demux/3 -> Scope2/3, Transfer Fcn3/1
  MATLAB Function/1(Dk) -> Demux/1, y/1
  Transfer Fcn2/1 -> Scope1/1
  Transfer Fcn1/1 -> Scope1/2
  Transfer Fcn3/1 -> Scope1/3
  "U "/1 -> Store 10 step1/1("Input ")
  xk/1 -> MATLAB Function/1(xk)
  Store 10 step1/1(Uk) -> Mux/1
  Store 10 step3/1(Uk) -> Mux/2
  Mux/1 -> MATLAB Function/3(Uk)
  Store 10 step2/2(Xk_delay 10) -> Store 10 step4/1("Input ")
  Store 10 step4/1(Xk) -> Mux1/2
  Store 10 step2/1(Xk) -> Mux1/1
  Mux1/1 -> MATLAB Function/2(X_sensor)
  Store 10 step1/2(Uk delay 10) -> Store 10 step3/1("Input ")

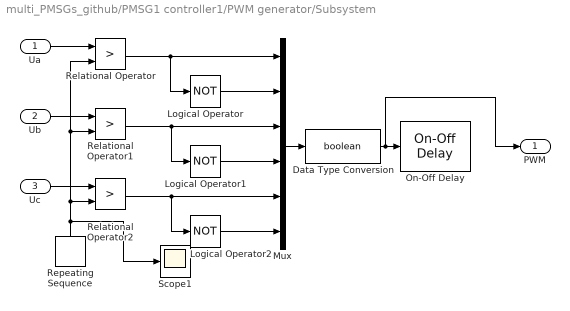
== system multi_PMSGs_github/PMSG1 controller1/PWM generator/Subsystem ==
  Ua : Inport
  Ub : Inport  Port=2
  Uc : Inport  Port=3
  Data Type Conversion : DataTypeConversion  OutDataTypeStr=boolean  SaturateOnIntegerOverflow=off  RndMeth=Floor
  Logical Operator : Logic  Operator=NOT  AllPortsSameDT=off  OutDataTypeStr=boolean
  Logical Operator1 : Logic  Operator=NOT  AllPortsSameDT=off  OutDataTypeStr=boolean
  Logical Operator2 : Logic  Operator=NOT  AllPortsSameDT=off  OutDataTypeStr=boolean
  Mux : Mux  Inputs=6
  On-Off Delay : eeGeneralControl/On-Off Delay  LabelModeActiveChoice=Discrete  Td_on=2e-6  Td_off=0  IC=0  Ts=2e-6
      settings: LibrarySourceBlock=ee_sl_lib/General Control/On-Off Delay
  Relational Operator : RelationalOperator  Operator=>  OutDataTypeStr=boolean  RndMeth=Simplest  InputSameDT=off
  Relational Operator1 : RelationalOperator  Operator=>  OutDataTypeStr=boolean  RndMeth=Simplest  InputSameDT=off
  Relational Operator2 : RelationalOperator  Operator=>  OutDataTypeStr=boolean  RndMeth=Simplest  InputSameDT=off
  Repeating Sequence : simulink/Sources/Repeating Sequence  rep_seq_t="[0  (1e-4)/2 1e-4]"  rep_seq_y=[-1 1 -1]
  Scope1 : Scope
  PWM : Outport
  wires:
  Ua/1 -> Relational Operator/1
  Ub/1 -> Relational Operator1/1
  Uc/1 -> Relational Operator2/1
  Repeating Sequence/1 -> Scope1/1, Relational Operator/2, Relational Operator1/2, Relational Operator2/2
  Logical Operator/1 -> Mux/2
  Relational Operator/1 -> Logical Operator/1, Mux/1
  Relational Operator1/1 -> Logical Operator1/1, Mux/3
  Logical Operator1/1 -> Mux/4
  Relational Operator2/1 -> Logical Operator2/1, Mux/5
  Logical Operator2/1 -> Mux/6
  Mux/1 -> Data Type Conversion/1
  Data Type Conversion/1 -> PWM/1, On-Off Delay/1

== system multi_PMSGs_github/PMSG1 controller/MHE/MHE1/Store 10 step1 ==
  "Input " : Inport
  Delay : Delay  DelayLength=1
  Delay1 : Delay
  Delay2 : Delay  DelayLength=3
  Delay3 : Delay  DelayLength=4
  Delay4 : Delay  DelayLength=5
  Delay5 : Delay  DelayLength=6
  Delay6 : Delay  DelayLength=7
  Delay7 : Delay  DelayLength=8
  Delay8 : Delay  DelayLength=9
  Mux : Mux  Inputs=10
  Uk : Outport
  Uk delay 10 : Outport  Port=2
  wires:
  Delay2/1 -> Mux/4
  Delay8/1 -> Uk delay 10/1, Mux/10
  "Input "/1 -> Mux/1, Delay/1, Delay1/1, Delay2/1, Delay3/1, Delay4/1, Delay5/1, Delay6/1, Delay7/1, Delay8/1
  Delay6/1 -> Mux/8
  Delay4/1 -> Mux/6
  Delay/1 -> Mux/2
  Delay5/1 -> Mux/7
  Delay3/1 -> Mux/5
  Delay1/1 -> Mux/3
  Mux/1 -> Uk/1
  Delay7/1 -> Mux/9

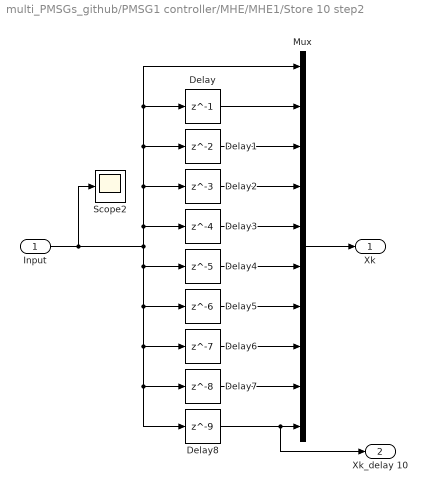
== system multi_PMSGs_github/PMSG1 controller/MHE/MHE1/Store 10 step2 ==
  "Input " : Inport
  Delay : Delay  DelayLength=1
  Delay1 : Delay
  Delay2 : Delay  DelayLength=3
  Delay3 : Delay  DelayLength=4
  Delay4 : Delay  DelayLength=5
  Delay5 : Delay  DelayLength=6
  Delay6 : Delay  DelayLength=7
  Delay7 : Delay  DelayLength=8
  Delay8 : Delay  DelayLength=9
  Mux : Mux  Inputs=10
  Scope2 : Scope
  Xk : Outport
  Xk_delay 10 : Outport  Port=2
  wires:
  Delay2/1 -> Mux/4
  Delay8/1 -> Xk_delay 10/1, Mux/10
  "Input "/1 -> Scope2/1, Mux/1, Delay/1, Delay1/1, Delay2/1, Delay3/1, Delay4/1, Delay5/1, Delay6/1, Delay7/1, Delay8/1
  Delay6/1 -> Mux/8
  Delay4/1 -> Mux/6
  Delay/1 -> Mux/2
  Delay5/1 -> Mux/7
  Delay3/1 -> Mux/5
  Delay1/1 -> Mux/3
  Mux/1 -> Xk/1
  Delay7/1 -> Mux/9

== system multi_PMSGs_github/PMSG1 controller/MHE/MHE1/Store 10 step3 ==
  "Input " : Inport
  Delay : Delay  DelayLength=1
  Delay1 : Delay
  Delay2 : Delay  DelayLength=3
  Delay3 : Delay  DelayLength=4
  Delay4 : Delay  DelayLength=5
  Delay5 : Delay  DelayLength=6
  Delay6 : Delay  DelayLength=7
  Delay7 : Delay  DelayLength=8
  Delay8 : Delay  DelayLength=9
  Mux : Mux  Inputs=10
  Uk : Outport
  wires:
  Delay2/1 -> Mux/4
  Delay8/1 -> Mux/10
  "Input "/1 -> Mux/1, Delay/1, Delay1/1, Delay2/1, Delay3/1, Delay4/1, Delay5/1, Delay6/1, Delay7/1, Delay8/1
  Delay6/1 -> Mux/8
  Delay4/1 -> Mux/6
  Delay/1 -> Mux/2
  Delay5/1 -> Mux/7
  Delay3/1 -> Mux/5
  Delay1/1 -> Mux/3
  Mux/1 -> Uk/1
  Delay7/1 -> Mux/9

== system multi_PMSGs_github/PMSG1 controller/MHE/MHE1/Store 10 step4 ==
  "Input " : Inport
  Delay : Delay  DelayLength=1
  Delay1 : Delay
  Delay2 : Delay  DelayLength=3
  Delay3 : Delay  DelayLength=4
  Delay4 : Delay  DelayLength=5
  Delay5 : Delay  DelayLength=6
  Delay6 : Delay  DelayLength=7
  Delay7 : Delay  DelayLength=8
  Delay8 : Delay  DelayLength=9
  Mux : Mux  Inputs=10
  Scope2 : Scope
  Xk : Outport
  wires:
  Delay2/1 -> Mux/4
  Delay8/1 -> Mux/10
  "Input "/1 -> Scope2/1, Mux/1, Delay/1, Delay1/1, Delay2/1, Delay3/1, Delay4/1, Delay5/1, Delay6/1, Delay7/1, Delay8/1
  Delay6/1 -> Mux/8
  Delay4/1 -> Mux/6
  Delay/1 -> Mux/2
  Delay5/1 -> Mux/7
  Delay3/1 -> Mux/5
  Delay1/1 -> Mux/3
  Mux/1 -> Xk/1
  Delay7/1 -> Mux/9

== system multi_PMSGs_github/PMSG1 controller1/MHE/MHE1/Store 10 step1 ==
  "Input " : Inport
  Delay : Delay  DelayLength=1
  Delay1 : Delay
  Delay2 : Delay  DelayLength=3
  Delay3 : Delay  DelayLength=4
  Delay4 : Delay  DelayLength=5
  Delay5 : Delay  DelayLength=6
  Delay6 : Delay  DelayLength=7
  Delay7 : Delay  DelayLength=8
  Delay8 : Delay  DelayLength=9
  Mux : Mux  Inputs=10
  Uk : Outport
  Uk delay 10 : Outport  Port=2
  wires:
  Delay2/1 -> Mux/4
  Delay8/1 -> Uk delay 10/1, Mux/10
  "Input "/1 -> Mux/1, Delay/1, Delay1/1, Delay2/1, Delay3/1, Delay4/1, Delay5/1, Delay6/1, Delay7/1, Delay8/1
  Delay6/1 -> Mux/8
  Delay4/1 -> Mux/6
  Delay/1 -> Mux/2
  Delay5/1 -> Mux/7
  Delay3/1 -> Mux/5
  Delay1/1 -> Mux/3
  Mux/1 -> Uk/1
  Delay7/1 -> Mux/9

== system multi_PMSGs_github/PMSG1 controller1/MHE/MHE1/Store 10 step2 ==
  "Input " : Inport
  Delay : Delay  DelayLength=1
  Delay1 : Delay
  Delay2 : Delay  DelayLength=3
  Delay3 : Delay  DelayLength=4
  Delay4 : Delay  DelayLength=5
  Delay5 : Delay  DelayLength=6
  Delay6 : Delay  DelayLength=7
  Delay7 : Delay  DelayLength=8
  Delay8 : Delay  DelayLength=9
  Mux : Mux  Inputs=10
  Scope2 : Scope
  Xk : Outport
  Xk_delay 10 : Outport  Port=2
  wires:
  Delay2/1 -> Mux/4
  Delay8/1 -> Xk_delay 10/1, Mux/10
  "Input "/1 -> Scope2/1, Mux/1, Delay/1, Delay1/1, Delay2/1, Delay3/1, Delay4/1, Delay5/1, Delay6/1, Delay7/1, Delay8/1
  Delay6/1 -> Mux/8
  Delay4/1 -> Mux/6
  Delay/1 -> Mux/2
  Delay5/1 -> Mux/7
  Delay3/1 -> Mux/5
  Delay1/1 -> Mux/3
  Mux/1 -> Xk/1
  Delay7/1 -> Mux/9

== system multi_PMSGs_github/PMSG1 controller1/MHE/MHE1/Store 10 step3 ==
  "Input " : Inport
  Delay : Delay  DelayLength=1
  Delay1 : Delay
  Delay2 : Delay  DelayLength=3
  Delay3 : Delay  DelayLength=4
  Delay4 : Delay  DelayLength=5
  Delay5 : Delay  DelayLength=6
  Delay6 : Delay  DelayLength=7
  Delay7 : Delay  DelayLength=8
  Delay8 : Delay  DelayLength=9
  Mux : Mux  Inputs=10
  Uk : Outport
  wires:
  Delay2/1 -> Mux/4
  Delay8/1 -> Mux/10
  "Input "/1 -> Mux/1, Delay/1, Delay1/1, Delay2/1, Delay3/1, Delay4/1, Delay5/1, Delay6/1, Delay7/1, Delay8/1
  Delay6/1 -> Mux/8
  Delay4/1 -> Mux/6
  Delay/1 -> Mux/2
  Delay5/1 -> Mux/7
  Delay3/1 -> Mux/5
  Delay1/1 -> Mux/3
  Mux/1 -> Uk/1
  Delay7/1 -> Mux/9

== system multi_PMSGs_github/PMSG1 controller1/MHE/MHE1/Store 10 step4 ==
  "Input " : Inport
  Delay : Delay  DelayLength=1
  Delay1 : Delay
  Delay2 : Delay  DelayLength=3
  Delay3 : Delay  DelayLength=4
  Delay4 : Delay  DelayLength=5
  Delay5 : Delay  DelayLength=6
  Delay6 : Delay  DelayLength=7
  Delay7 : Delay  DelayLength=8
  Delay8 : Delay  DelayLength=9
  Mux : Mux  Inputs=10
  Scope2 : Scope
  Xk : Outport
  wires:
  Delay2/1 -> Mux/4
  Delay8/1 -> Mux/10
  "Input "/1 -> Scope2/1, Mux/1, Delay/1, Delay1/1, Delay2/1, Delay3/1, Delay4/1, Delay5/1, Delay6/1, Delay7/1, Delay8/1
  Delay6/1 -> Mux/8
  Delay4/1 -> Mux/6
  Delay/1 -> Mux/2
  Delay5/1 -> Mux/7
  Delay3/1 -> Mux/5
  Delay1/1 -> Mux/3
  Mux/1 -> Xk/1
  Delay7/1 -> Mux/9

== matlab function multi_PMSGs_github/PMSG1 controller/Compensation law/MATLAB Function ==
  data: w input; u_com output; K1 input; K2 input; K3 input; X input; X_hat input; w_ref input
function u_com = compensation (w,K1,K2,K3,X,X_hat,w_ref)
Rs = 1.3;
phi_f = 0.4;
L = 0.75e-3;
J = 0.0008;
B = 0.00001;
p = 2;
Ts = 1e-6;

A = [-Rs/L,-p*(X(3)-w_ref),-p*phi_f/L;
     p*(X(3)-w_ref),-Rs/L,0;
     1.5*p*phi_f/J,0,-B/J];
Bc = [1/L 0 0;
      0 1/L 0;
      0 0 -1/J];
A_hat = [-Rs/L,-p*(X_hat(3)-w_ref),-p*phi_f/L;
     p*(X_hat(3)-w_ref),-Rs/L,0;
     1.5*p*phi_f/J,0,-B/J];
A_d = Ts*A+eye(size(A,1)); 
Bc_d = Ts*Bc;
K = diag([K1,K2,K3]);
u_com = -(Bc_d^-1)*A_d*w-(Bc_d^-1)*K*w;
u_com = -(Bc^-1)*(-A-K)*w;
u_com = -Bc^-1*(A_hat*X_hat-A*X-w-K*(X-X_hat));

== matlab function multi_PMSGs_github/PMSG1 controller/MHE/MATLAB Function1 ==
  data: xk input; u input; xk_dot output
function xk_dot = model(xk,u)

Rs = 1.3;
phi_f = 0.4;
L = 0.75e-3;
J = 0.0008;
B = 0.00001;
p = 2;
Ts = 1e-6;
%%预测周期
%N = 20;


A = [-Rs/L,-p*(xk(3)),-p*phi_f/L;
     p*(xk(3)),-Rs/L,0;
     1.5*p*phi_f/J,0,-B/J];
Bc = [1/L 0 0;
      0 1/L 0;
      0 0 -1/J];
A_d = Ts*A+eye(size(A,1)); 
Bc_d = Ts*Bc;
xk_dot = A_d*xk+Bc_d*u;

== matlab function multi_PMSGs_github/PMSG1 controller/MHE/MHE1/MATLAB Function ==
  data: xk input; Dk output size=3; X_sensor input; Uk input; x_ref input
function Dk = MHE(xk,X_sensor,Uk,x_ref)
iq = xk(1);
id = xk(2);
w = xk(3);
w_ref = x_ref(3);
Rs = 1.3;
phi_f = 0.4;
L = 0.75e-3;
J = 0.0008;
B = 0.00001;
p = 2;
Ts = 1e-6;
N=20;
A = [-Rs/L,-p*(w),-p*phi_f/L;
     p*(w),-Rs/L,0;
     1.5*p*phi_f/J,0,-B/J];
Bc = [1/L 0 0;
      0 1/L 0;
      0 0 -1/J];
A_d = Ts*A+eye(size(A,1));
Bc_d = Ts*Bc;
n = size(A_d,1);
p = size(Bc,2);
tmp = eye(n);
C = zeros(N*n,N*p);
E = zeros(N*n,N*p);
M = [eye(n);zeros((N-1)*n,n)];
I = eye(n);
for i = 1:N-1
    rows = i*n+(1:n);
    C(rows,:) = [tmp*Bc_d, C(rows-n, 1:end-p)];
    E(rows,:) = [tmp*I, E(rows-n, 1:end-p)];
    tmp = A_d*tmp;
    M(rows, :) = tmp;
end
lb1 = zeros(1,N)-20;
lb2 = zeros(1,N)-20;
lb3 = zeros(1,N)-20;
ub1 = zeros(1,N)+20;
ub2 = zeros(1,N)+20;
ub3 = zeros(1,N)+20;
lb = [lb1;lb2;lb3];
ub = [ub1;ub2;ub3];
%%权重系数
Q = [1 0 0;
     0 1 0;
     0 0 10];
P=[291	0	0;
0	175	0;
0	0	13000;];

R = [0.01 0 0;
     0 0.01 0;
     0 0 0.01];

Q_bar = kron(eye(N-1),Q);
Q_bar = blkdiag(Q_bar,P);
R_bar = kron(eye(N),R);

H = xk.'*M.'*Q_bar*E+Uk.'*C.'*Q_bar*E-X_sensor.'*Q_bar*E;
L = E.'*Q_bar*E+R_bar;
% H = xk.'*M.'*Q_bar+Uk.'*C.'*Q_bar-X_sensor.'*Q_bar;
% L = Q_bar+R_bar;
options = optimoptions('quadprog','Algorithm','active-set');
D_K = quadprog(L,H,[],[],[],[],lb,ub,zeros(size(L,2),1),options);
%Dk = D_K(end-2:end);
Dk = D_K(1:3);

== matlab function multi_PMSGs_github/PMSG1 controller1/Compensation law/MATLAB Function ==
  data: w input; u_com output; K1 input; K2 input; K3 input; X input; X_hat input; w_ref input
function u_com = compensation (w,K1,K2,K3,X,X_hat,w_ref)
Rs = 1.3;
phi_f = 0.4;
L = 0.75e-3;
J = 0.0008;
B = 0.00001;
p = 2;
Ts = 1e-6;

A = [-Rs/L,-p*(X(3)-w_ref),-p*phi_f/L;
     p*(X(3)-w_ref),-Rs/L,0;
     1.5*p*phi_f/J,0,-B/J];
Bc = [1/L 0 0;
      0 1/L 0;
      0 0 -1/J];
A_hat = [-Rs/L,-p*(X_hat(3)-w_ref),-p*phi_f/L;
     p*(X_hat(3)-w_ref),-Rs/L,0;
     1.5*p*phi_f/J,0,-B/J];
A_d = Ts*A+eye(size(A,1)); 
Bc_d = Ts*Bc;
K = diag([K1,K2,K3]);
u_com = -(Bc_d^-1)*A_d*w-(Bc_d^-1)*K*w;
u_com = -(Bc^-1)*(-A-K)*w;
u_com = -Bc^-1*(A_hat*X_hat-A*X-w-K*(X-X_hat));

== matlab function multi_PMSGs_github/PMSG1 controller1/MHE/MATLAB Function1 ==
  data: xk input; u input; xk_dot output
function xk_dot = model(xk,u)

Rs = 1.3;
phi_f = 0.4;
L = 0.75e-3;
J = 0.0008;
B = 0.00001;
p = 2;
Ts = 1e-6;
%%预测周期
%N = 20;


A = [-Rs/L,-p*(xk(3)),-p*phi_f/L;
     p*(xk(3)),-Rs/L,0;
     1.5*p*phi_f/J,0,-B/J];
Bc = [1/L 0 0;
      0 1/L 0;
      0 0 -1/J];
A_d = Ts*A+eye(size(A,1)); 
Bc_d = Ts*Bc;
xk_dot = A_d*xk+Bc_d*u;

== matlab function multi_PMSGs_github/PMSG1 controller1/MHE/MHE1/MATLAB Function ==
  data: xk input; Dk output size=3; X_sensor input; Uk input; x_ref input
function Dk = MHE(xk,X_sensor,Uk,x_ref)
iq = xk(1);
id = xk(2);
w = xk(3);
w_ref = x_ref(3);
Rs = 1.3;
phi_f = 0.4;
L = 0.75e-3;
J = 0.0008;
B = 0.00001;
p = 2;
Ts = 1e-6;
N=20;
A = [-Rs/L,-p*(w),-p*phi_f/L;
     p*(w),-Rs/L,0;
     1.5*p*phi_f/J,0,-B/J];
Bc = [1/L 0 0;
      0 1/L 0;
      0 0 -1/J];
A_d = Ts*A+eye(size(A,1));
Bc_d = Ts*Bc;
n = size(A_d,1);
p = size(Bc,2);
tmp = eye(n);
C = zeros(N*n,N*p);
E = zeros(N*n,N*p);
M = [eye(n);zeros((N-1)*n,n)];
I = eye(n);
for i = 1:N-1
    rows = i*n+(1:n);
    C(rows,:) = [tmp*Bc_d, C(rows-n, 1:end-p)];
    E(rows,:) = [tmp*I, E(rows-n, 1:end-p)];
    tmp = A_d*tmp;
    M(rows, :) = tmp;
end
lb1 = zeros(1,N)-20;
lb2 = zeros(1,N)-20;
lb3 = zeros(1,N)-20;
ub1 = zeros(1,N)+20;
ub2 = zeros(1,N)+20;
ub3 = zeros(1,N)+20;
lb = [lb1;lb2;lb3];
ub = [ub1;ub2;ub3];
%%权重系数
Q = [1 0 0;
     0 1 0;
     0 0 10];
P=[291	0	0;
0	175	0;
0	0	13000;];

R = [0.01 0 0;
     0 0.01 0;
     0 0 0.01];

Q_bar = kron(eye(N-1),Q);
Q_bar = blkdiag(Q_bar,P);
R_bar = kron(eye(N),R);

H = xk.'*M.'*Q_bar*E+Uk.'*C.'*Q_bar*E-X_sensor.'*Q_bar*E;
L = E.'*Q_bar*E+R_bar;
% H = xk.'*M.'*Q_bar+Uk.'*C.'*Q_bar-X_sensor.'*Q_bar;
% L = Q_bar+R_bar;
options = optimoptions('quadprog','Algorithm','active-set');
D_K = quadprog(L,H,[],[],[],[],lb,ub,zeros(size(L,2),1),options);
%Dk = D_K(end-2:end);
Dk = D_K(1:3);

== matlab function multi_PMSGs_github/PMSG1 controller1/MPC/MPC controller  ==
  data: id input; iq input; w input; w_ref input; iq_ref input; ud output; uq output; TL output; Q input; R input; N input; K input; x_ref_dot input; Ts input; d input
function [ud,uq,TL] = MPC(id,iq,w,w_ref,iq_ref,Q,R,N,K,x_ref_dot,Ts,d)
Rs = 1.3;
phi_f = 0.4;
L = 0.75e-3;
id_ref = 0;
J = 0.0008;
B = 0.00001;
p = 2;
%Ts = 1e-5;
%%预测周期
%N = 20;
X = [iq-iq_ref;id-id_ref;w-w_ref];
x_ref = [iq_ref;id_ref;w_ref];
A = [-Rs/L,-p*(w-w_ref),-p*phi_f/L;
     p*(w-w_ref),-Rs/L,0;
     1.5*p*phi_f/J,0,-B/J];
Bc = [1/L 0 0;
      0 1/L 0;
      0 0 -1/J];
A_d = Ts*A+eye(size(A,1));
Bc_d = Ts*Bc;
D = kron(ones(N,1),d);
%%权重系数
% Q = [30 0 0;
%      0 30 0;
%      0 0 5];
F = eye(3);

% R = [0.01 0 0;
%      0 0.01 0;
%      0 0 0.001];

n = size(A_d,1);
p = size(Bc,2);
%q = size(D,2);
Alpha = Ts*(x_ref_dot-K*x_ref);
% Alpha = x_ref_dot-K*x_ref;
Beta = eye(size(A,1))-Ts*K;
% Beta = K;
M = [eye(n);zeros((N+1)*n,n)];
C = zeros((N+2)*n,N*p);
E = zeros((N+2)*n,N*p);
S = [zeros((N+1)*n,1);Alpha];
A_ineq = [Bc_d,zeros(n,(N-1)*p);zeros((N-1)*n,(N)*p)];
b_ineq = zeros((N)*n,1);
%D_bar = zeros((N+1)*n,q);
tmp = eye(n);
lb1 = zeros(1,N)-600;
lb2 = zeros(1,N)-600;
lb3 = zeros(1,N)-300;
ub1 = zeros(1,N)+600;
ub2 = zeros(1,N)+600;
ub3 = zeros(1,N)+300;
lb = [lb1;lb2;lb3];
ub = [ub1;ub2;ub3];
%state constrain
% e_iq,e_id,e_w
lb_s = [-100;-10;-10];
ub_s = [100;10;10];
Ak = eye(3)-Ts*K;
 Ak = [-0.982666666666667	0	0;
0	-0.982666666666667	0;
0	0	-1];
Xf = (-Ak)*[lb_s,ub_s];

lb_state = [kron(ones(N-1,1),lb_s);Xf(:,1)];
ub_state = [kron(ones(N-1,1),ub_s);Xf(:,2)];

%lb_state = zeros((N)*size(A_d,1),1)-20;
%ub_state = zeros((N)*size(A_d,1),1)+40;
%lb = [-600,-600,-600];
%ub = [600,600,0];
%%更新M和C
for i = 1:N
    rows = i*n+(1:n);
    C(rows,:) = [tmp*Bc_d, C(rows-n, 1:end-p)];
    E(rows,:) = [tmp, E(rows-n, 1:end-p)];
    tmp = A_d*tmp; 
    M(rows, :) = tmp;
    col = (i-1)*n+(1:n);
    %tmp = A_d*tmp;
    A_ineq(rows-n, :) = [(tmp*Bc_d), A_ineq(rows-n, 1:end-p)];   
    b_ineq(col, :) = tmp*X;    
end
A_ineq=[A_ineq;-A_ineq];
b_ineq=[ub_state-b_ineq;-lb_state+b_ineq];
P=[291	0	0;
0	17500	0;
0	0	130000000;];
%P = eye(3);
%%定义Q_bar和R_bar
M((N+1)*n+(1:n),:) = Beta*M(N*n+(1:n),:);
C((N+1)*n+(1:n),:) = Beta*C(N*n+(1:n),:);
Q_bar = kron(eye(N+1),Q);
Q_bar = blkdiag(Q_bar,P);
R_bar = kron(eye(N),R);

%%计算G,E,H
H = C'*Q_bar*C + R_bar;
E = C'*Q_bar*M*X+C'*Q_bar*S+C'*Q_bar*E*D; 
E = C'*Q_bar*M*X+C'*Q_bar*S ;

options = optimoptions('quadprog','Algorithm','active-set');
U_K = quadprog(H,E,A_ineq,b_ineq,[],[],lb,ub,zeros(size(H,2),1),options);
%U_K = quadprog(H,E,[],[],[],[],lb,ub,zeros(size(H,2),1),options);
u_k = U_K(1:p,1);

uq = u_k(1);
ud = u_k(2);
TL = u_k(3);
end

== matlab function multi_PMSGs_github/PMSG1 controller/MPC/MPC controller  ==
  data: id input; iq input; w input; w_ref input; iq_ref input; ud output; uq output; TL output; Q input; R input; N input; K input; x_ref_dot input; Ts input; d input
function [ud,uq,TL] = MPC(id,iq,w,w_ref,iq_ref,Q,R,N,K,x_ref_dot,Ts,d)
Rs = 1.3;
phi_f = 0.4;
L = 0.75e-3;
id_ref = 0;
J = 0.0008;
B = 0.00001;
p = 2;
%Ts = 1e-5;
%%预测周期
%N = 20;
X = [iq-iq_ref;id-id_ref;w-w_ref];
x_ref = [iq_ref;id_ref;w_ref];
A = [-Rs/L,-p*(w-w_ref),-p*phi_f/L;
     p*(w-w_ref),-Rs/L,0;
     1.5*p*phi_f/J,0,-B/J];
Bc = [1/L 0 0;
      0 1/L 0;
      0 0 -1/J];
A_d = Ts*A+eye(size(A,1));
Bc_d = Ts*Bc;
D = kron(ones(N,1),d);
%%权重系数
% Q = [30 0 0;
%      0 30 0;
%      0 0 5];
F = eye(3);

% R = [0.01 0 0;
%      0 0.01 0;
%      0 0 0.001];

n = size(A_d,1);
p = size(Bc,2);
%q = size(D,2);
Alpha = Ts*(x_ref_dot-K*x_ref);
% Alpha = x_ref_dot-K*x_ref;
Beta = eye(size(A,1))-Ts*K;
% Beta = K;
M = [eye(n);zeros((N+1)*n,n)];
C = zeros((N+2)*n,N*p);
E = zeros((N+2)*n,N*p);
S = [zeros((N+1)*n,1);Alpha];
A_ineq = [Bc_d,zeros(n,(N-1)*p);zeros((N-1)*n,(N)*p)];
b_ineq = zeros((N)*n,1);
%D_bar = zeros((N+1)*n,q);
tmp = eye(n);
lb1 = zeros(1,N)-600;
lb2 = zeros(1,N)-600;
lb3 = zeros(1,N)-300;
ub1 = zeros(1,N)+600;
ub2 = zeros(1,N)+600;
ub3 = zeros(1,N)+300;
lb = [lb1;lb2;lb3];
ub = [ub1;ub2;ub3];
%state constrain
% e_iq,e_id,e_w
lb_s = [-100;-10;-10];
ub_s = [100;10;10];
Ak = eye(3)-Ts*K;
 Ak = [-0.982666666666667	0	0;
0	-0.982666666666667	0;
0	0	-1];
Xf = (-Ak)*[lb_s,ub_s];

lb_state = [kron(ones(N-1,1),lb_s);Xf(:,1)];
ub_state = [kron(ones(N-1,1),ub_s);Xf(:,2)];

%lb_state = zeros((N)*size(A_d,1),1)-20;
%ub_state = zeros((N)*size(A_d,1),1)+40;
%lb = [-600,-600,-600];
%ub = [600,600,0];
%%更新M和C
for i = 1:N
    rows = i*n+(1:n);
    C(rows,:) = [tmp*Bc_d, C(rows-n, 1:end-p)];
    E(rows,:) = [tmp, E(rows-n, 1:end-p)];
    tmp = A_d*tmp; 
    M(rows, :) = tmp;
    col = (i-1)*n+(1:n);
    %tmp = A_d*tmp;
    A_ineq(rows-n, :) = [(tmp*Bc_d), A_ineq(rows-n, 1:end-p)];   
    b_ineq(col, :) = tmp*X;    
end
A_ineq=[A_ineq;-A_ineq];
b_ineq=[ub_state-b_ineq;-lb_state+b_ineq];
P=[291	0	0;
0	17500	0;
0	0	130000000;];
%P = eye(3);
%%定义Q_bar和R_bar
M((N+1)*n+(1:n),:) = Beta*M(N*n+(1:n),:);
C((N+1)*n+(1:n),:) = Beta*C(N*n+(1:n),:);
Q_bar = kron(eye(N+1),Q);
Q_bar = blkdiag(Q_bar,P);
R_bar = kron(eye(N),R);

%%计算G,E,H
H = C'*Q_bar*C + R_bar;
E = C'*Q_bar*M*X+C'*Q_bar*S+C'*Q_bar*E*D; 
E = C'*Q_bar*M*X+C'*Q_bar*S ;

options = optimoptions('quadprog','Algorithm','active-set');
U_K = quadprog(H,E,A_ineq,b_ineq,[],[],lb,ub,zeros(size(H,2),1),options);
%U_K = quadprog(H,E,[],[],[],[],lb,ub,zeros(size(H,2),1),options);
u_k = U_K(1:p,1);

uq = u_k(1);
ud = u_k(2);
TL = u_k(3);
end
